simulink library "ESTS_SLA"  (R2024b)
settings: Solver=VariableStepAuto  StartTime=0.0  StopTime=10.0  RelTol=1e-3
undefined symbols (not defined in the file): p_dt_s
libraries: sharedTrackingLibrary x1, simulink_extras x1
settings Model: Creator=blatak  LastModifiedBy=blatak
settings ModelReferenceCC: EnableRefExpFcnMdlSchedulingChecks=on
settings RTWCC: GPUComputeCapability=3.5

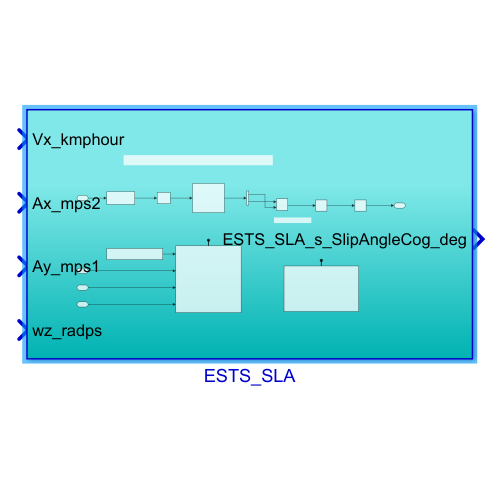
[thumbnail: Simulink's stored preview of the top-level diagram]
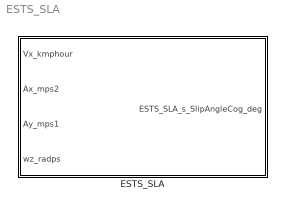
== system ESTS_SLA ==
  ESTS_SLA : Subsystem

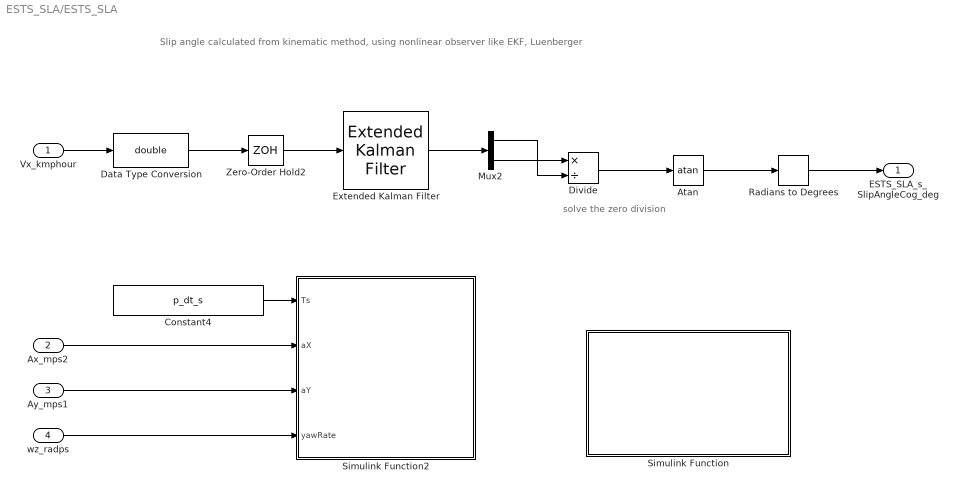
== system ESTS_SLA/ESTS_SLA ==
  note: solve the zero division
  note: Slip angle calculated from kinematic method, using nonlinear observer like EKF, Luenberger
  Vx_kmphour : Inport
  Ax_mps2 : Inport  Port=2
  Ay_mps1 : Inport  Port=3
  wz_radps : Inport  Port=4
  Atan : Trigonometry  Operator=atan
  Constant4 : Constant  Value=p_dt_s
  Data Type Conversion : DataTypeConversion  OutDataTypeStr=double  SaturateOnIntegerOverflow=off  RndMeth=Floor
  Divide : Product  Inputs=*/
  Extended Kalman Filter : sharedTrackingLibrary/Extended Kalman Filter  StateTransitionFcn=fcnVehicleModel  HasStateTransitionJacobianFcn=off  HasAdditiveProcessNoise=Additive  ProcessNoise=diag([1e-3, 1e-3])  HasTimeVaryingProcessNoise=off  HasStateTransitionFcnExtraArgument=0  InitialState=[0 0]  InitialStateCovariance=1e-6  MeasurementFcn1=fcnMeasurementVx  HasMeasurementJacobianFcn1=off  HasMeasurementEnablePort1=off  HasAdditiveMeasurementNoise1=Additive  MeasurementNoise1=1e-4  HasTimeVaryingMeasurementNoise1=off  HasMeasurementFcnExtraArgument1=0  HasMeasurementWrapping1=off  MeasurementFcn2=myMeasurementFcn  HasMeasurementJacobianFcn2=off  HasMeasurementEnablePort2=off  HasAdditiveMeasurementNoise2=Additive  MeasurementNoise2=1  HasTimeVaryingMeasurementNoise2=off  HasMeasurementFcnExtraArgument2=0  HasMeasurementWrapping2=off  MeasurementFcn3=myMeasurementFcn  HasMeasurementJacobianFcn3=off  HasMeasurementEnablePort3=off  HasAdditiveMeasurementNoise3=Additive  MeasurementNoise3=1  HasTimeVaryingMeasurementNoise3=off  HasMeasurementFcnExtraArgument3=0  HasMeasurementWrapping3=off  MeasurementFcn4=myMeasurementFcn  HasMeasurementJacobianFcn4=off  HasMeasurementEnablePort4=off  HasAdditiveMeasurementNoise4=Additive  MeasurementNoise4=1  HasTimeVaryingMeasurementNoise4=off  HasMeasurementFcnExtraArgument4=0  HasMeasurementWrapping4=off  MeasurementFcn5=myMeasurementFcn  HasMeasurementJacobianFcn5=off  HasMeasurementEnablePort5=off  HasAdditiveMeasurementNoise5=Additive  MeasurementNoise5=1  HasTimeVaryingMeasurementNoise5=off  HasMeasurementFcnExtraArgument5=0  HasMeasurementWrapping5=off  EnableMultirate=off  StateTransitionFcnSampleTime=1  MeasurementFcn1SampleTime=1  MeasurementFcn2SampleTime=1  MeasurementFcn3SampleTime=1  MeasurementFcn4SampleTime=1  MeasurementFcn5SampleTime=1  UseCurrentEstimator=on  OutputStateCovariance=off  DataType=double  SampleTime=-1  NumberOfMeasurements=1
  Mux2 : Demux  Outputs=2
  Radians to Degrees : simulink_extras/Transformations/Radians to Degrees
  Simulink Function : Subsystem  TreatAsAtomicUnit=on
  Simulink Function2 : Subsystem  TreatAsAtomicUnit=on
  Zero-Order Hold2 : ZeroOrderHold  SampleTime=-1
  ESTS_SLA_s_SlipAngleCog_deg : Outport
  wires:
  wz_radps/1 -> Simulink Function2/4(yawRate)
  Ay_mps1/1 -> Simulink Function2/3(aY)
  Ax_mps2/1 -> Simulink Function2/2(aX)
  Vx_kmphour/1 -> Data Type Conversion/1
  Data Type Conversion/1 -> Zero-Order Hold2/1
  Zero-Order Hold2/1 -> Extended Kalman Filter/1
  Radians to Degrees/1 -> ESTS_SLA_s_SlipAngleCog_deg/1
  Divide/1 -> Atan/1
  Atan/1 -> Radians to Degrees/1
  Mux2/2 -> Divide/1
  Mux2/1 -> Divide/2
  Extended Kalman Filter/1 -> Mux2/1
  Constant4/1 -> Simulink Function2/1(Ts)

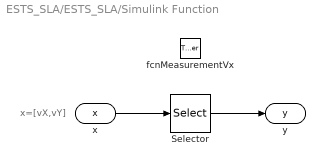
== system ESTS_SLA/ESTS_SLA/Simulink Function ==
  note: x=[vX,vY]
  fcnMeasurementVx : TriggerPort  TriggerType=function-call  IsSimulinkFunction=on  FunctionName=fcnMeasurementVx  FunctionVisibility=scoped  VariantControl=(inherit)
  Selector : Selector  InputPortWidth=2  IndexOptions=Index vector (dialog)  Indices=1  OutputSizes=1
  x : ArgIn  DisableCoverage=on  PortDimensions=2  ArgumentName=x
  y : ArgOut  DisableCoverage=on  ArgumentName=y
  wires:
  Selector/1 -> y/1
  x/1 -> Selector/1

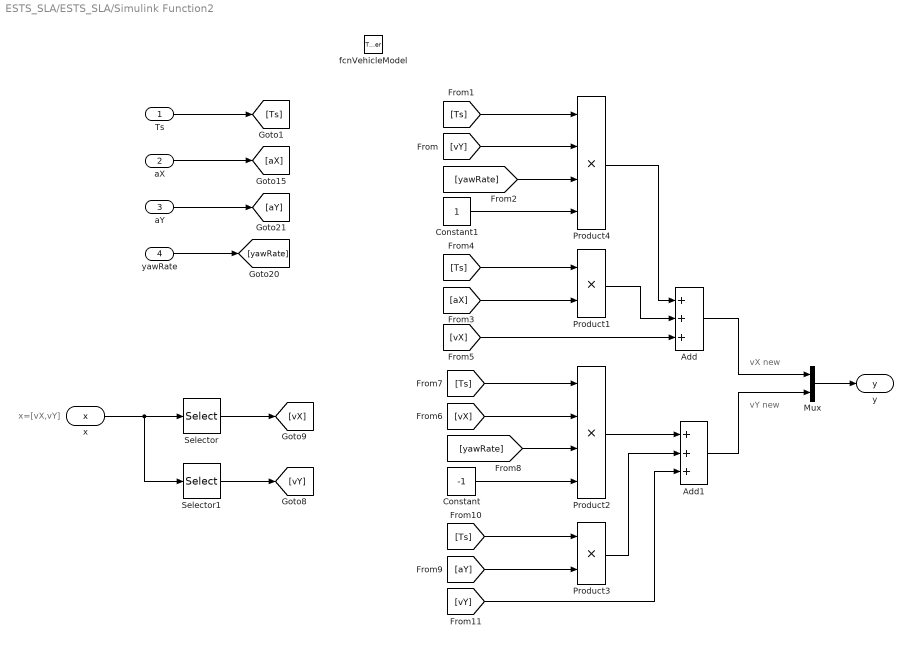
== system ESTS_SLA/ESTS_SLA/Simulink Function2 ==
  note: vY new
  note: x=[vX,vY]
  note: vX new
  Ts : Inport
  aX : Inport  Port=2
  aY : Inport  Port=3
  yawRate : Inport  Port=4
  fcnVehicleModel : TriggerPort  TriggerType=function-call  IsSimulinkFunction=on  FunctionName=fcnVehicleModel  FunctionVisibility=scoped  VariantControl=(inherit)
  Add : Sum  Inputs=+++
  Add1 : Sum  Inputs=+++
  Constant : Constant  Value=-1
  Constant1 : Constant
  Mux : Mux  Inputs=2
  Product1 : Product
  Product2 : Product  Inputs=4
  Product3 : Product
  Product4 : Product  Inputs=4
  Selector : Selector  InputPortWidth=2  IndexOptions=Index vector (dialog)  Indices=1  OutputSizes=1
  Selector1 : Selector  InputPortWidth=2  IndexOptions=Index vector (dialog)  Indices=2  OutputSizes=1
  x : ArgIn  DisableCoverage=on  PortDimensions=2  ArgumentName=x
  y : ArgOut  DisableCoverage=on  PortDimensions=2  ArgumentName=y
  wires:
  [Ts] -> Product4/1
  Add1/1 -> Mux/2
  Product1/1 -> Add/2
  Add/1 -> Mux/1
  Mux/1 -> y/1
  Product2/1 -> Add1/1
  [yawRate] -> Product4/3
  [vY] -> Add1/3
  [vX] -> Add/3
  [Ts] -> Product1/1
  Ts/1 -> [Ts]
  Constant1/1 -> Product4/4
  Constant/1 -> Product2/4
  [Ts] -> Product3/1
  [vX] -> Product2/2
  aY/1 -> [aY]
  Product3/1 -> Add1/2
  aX/1 -> [aX]
  [Ts] -> Product2/1
  [aX] -> Product1/2
  [yawRate] -> Product2/3
  yawRate/1 -> [yawRate]
  x/1 -> Selector/1, Selector1/1
  [vY] -> Product4/2
  Product4/1 -> Add/1
  [aY] -> Product3/2
  Selector/1 -> [vX]
  Selector1/1 -> [vY]
